simulink model "IBVSstereo"  (Simulink 10.0)
settings: Solver=ode45  StartTime=0.0  StopTime=30.0  RelTol=1e-3  EnableMultiTasking=on
undefined symbols (not defined in the file): coords, get, GetHMatrix, lc, p, rc, T0e_0, T0e_x, T0o, Telc, Terc
libraries: vs x31, simulink x3
settings Model: Creator=bhisma  LastModifiedBy=bhisma
settings DataIOCC: LimitDataPoints=on  SignalLoggingSaveFormat=ModelDataLogs  SignalLoggingName=sigsOut
settings OptimizationCC: BooleanDataType=off  LifeSpan=auto
settings DebuggingCC: SaveWithParameterizedLinksMsg=none  SignalResolutionControl=TryResolveAllWithWarning  MultiTaskDSMMsg=warning  MultiTaskCondExecSysMsg=none  SFUnexpectedBacktrackingDiag=error  SFNoUnconditionalDefaultTransitionDiag=error  SFExecutionAtInitializationDiag=warning  ArithmeticOperatorsInVariantConditions=error
settings HardwareCC: TargetUnknown=on
settings SFSimCC: SimUseLocalCustomCode=on  CustomCodeUndefinedFunction=FilterOut
settings RTWCC: RTWUseLocalCustomCode=on
settings CodeAppCC: StateflowObjectComments=off
settings GRTTargetCC: TargetLangStandard=C99 (ISO)

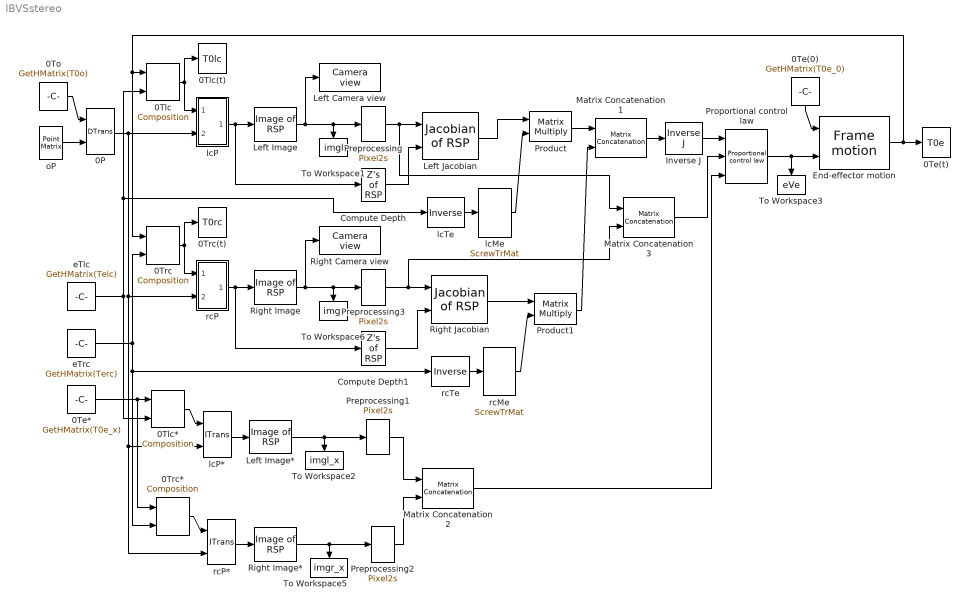
== system IBVSstereo ==
  0P : vs/Features/DTrans  SimViewingDevice=off  DataTypeOverride=UseLocalSettings  MinMaxOverflowLogging=UseLocalSettings
      settings: Permissions=ReadWrite  RTWFcnNameOpts=Auto  RTWFileNameOpts=Auto
  0Te(0) : Constant  Value=GetHMatrix(T0e_0)  VectorParams1D=off
  0Te(t) : ToWorkspace  VariableName=T0e  SaveFormat=Structure With Time  SampleTime=-1
  0Te* : Constant  Value=GetHMatrix(T0e_x)  VectorParams1D=off
  0Tlc : vs/Pose/Composition  SimViewingDevice=off  DataTypeOverride=UseLocalSettings  MinMaxOverflowLogging=UseLocalSettings
      settings: Permissions=ReadWrite  RTWFcnNameOpts=Auto  RTWFileNameOpts=Auto
  0Tlc(t) : ToWorkspace  VariableName=T0lc  SaveFormat=Structure With Time  SampleTime=-1
  0Tlc* : vs/Pose/Composition  SimViewingDevice=off  DataTypeOverride=UseLocalSettings  MinMaxOverflowLogging=UseLocalSettings
      settings: Permissions=ReadWrite  RTWFcnNameOpts=Auto  RTWFileNameOpts=Auto
  0To : Constant  Value=GetHMatrix(T0o)  VectorParams1D=off
  0Trc : vs/Pose/Composition  SimViewingDevice=off  DataTypeOverride=UseLocalSettings  MinMaxOverflowLogging=UseLocalSettings
      settings: Permissions=ReadWrite  RTWFcnNameOpts=Auto  RTWFileNameOpts=Auto
  0Trc(t) : ToWorkspace  VariableName=T0rc  SaveFormat=Structure With Time  SampleTime=-1
  0Trc* : vs/Pose/Composition  SimViewingDevice=off  DataTypeOverride=UseLocalSettings  MinMaxOverflowLogging=UseLocalSettings
      settings: Permissions=ReadWrite  RTWFcnNameOpts=Auto  RTWFileNameOpts=Auto
  Compute Depth : vs/Features/Z's of RSP  SimViewingDevice=off  DataTypeOverride=UseLocalSettings  MinMaxOverflowLogging=UseLocalSettings
      settings: Permissions=ReadWrite  RTWFcnNameOpts=Auto  RTWFileNameOpts=Auto
  Compute Depth1 : vs/Features/Z's of RSP  SimViewingDevice=off  DataTypeOverride=UseLocalSettings  MinMaxOverflowLogging=UseLocalSettings
      settings: Permissions=ReadWrite  RTWFcnNameOpts=Auto  RTWFileNameOpts=Auto
  End-effector motion : vs/Pose/Frame motion  SimViewingDevice=off  DataTypeOverride=UseLocalSettings  MinMaxOverflowLogging=UseLocalSettings
      settings: Permissions=ReadWrite  RTWFcnNameOpts=Auto  RTWFileNameOpts=Auto
  Inverse J : vs/Jacobian/Inverse J  SimViewingDevice=off  DataTypeOverride=UseLocalSettings  MinMaxOverflowLogging=UseLocalSettings
      settings: Permissions=ReadWrite  RTWFcnNameOpts=Auto  RTWFileNameOpts=Auto
  Left Camera view : vs/Camera/Camera view  ms=15  em=normal  umin=0  umax=get(lc,'hres')-1  vmin=0  vmax=get(lc,'vres')-1  st=-1
  Left Image : vs/Camera/Image of RSP  fu=get(lc,'fu')  fv=get(lc,'fv')  u0=get(lc,'u0')  v0=get(lc,'v0')
  Left Image* : vs/Camera/Image of RSP  fu=get(lc,'fu')  fv=get(lc,'fv')  u0=get(lc,'u0')  v0=get(lc,'v0')
  Left Jacobian : vs/Jacobian/Jacobian of RSP  SimViewingDevice=off  DataTypeOverride=UseLocalSettings  MinMaxOverflowLogging=UseLocalSettings
      settings: Permissions=ReadWrite  RTWFcnNameOpts=Auto  RTWFileNameOpts=Auto
  Matrix Concatenation1 : simulink/Math Operations/Matrix Concatenation  numInports=2  catMethod=Vertical
      settings: SourceProductName=Simulink  SourceProductBaseCode=SL
  Matrix Concatenation2 : simulink/Math Operations/Matrix Concatenation  numInports=2  catMethod=Vertical
      settings: SourceProductName=Simulink  SourceProductBaseCode=SL
  Matrix Concatenation3 : simulink/Math Operations/Matrix Concatenation  numInports=2  catMethod=Vertical
      settings: SourceProductName=Simulink  SourceProductBaseCode=SL
  Preprocessing : vs/Jacobian/Pixel2s  fu=get(lc,'fu')  fv=get(lc,'fv')  u0=get(lc,'u0')  v0=get(lc,'v0')
  Preprocessing1 : vs/Jacobian/Pixel2s  fu=get(lc,'fu')  fv=get(lc,'fv')  u0=get(lc,'u0')  v0=get(lc,'v0')
  Preprocessing2 : vs/Jacobian/Pixel2s  fu=get(rc,'fu')  fv=get(rc,'fv')  u0=get(rc,'u0')  v0=get(rc,'v0')
  Preprocessing3 : vs/Jacobian/Pixel2s  fu=get(rc,'fu')  fv=get(rc,'fv')  u0=get(rc,'u0')  v0=get(rc,'v0')
  Product : Product  Multiplication=Matrix(*)  SaturateOnIntegerOverflow=on  InputSameDT=on  OutDataTypeStr=Inherit: Same as first input
  Product1 : Product  Multiplication=Matrix(*)  SaturateOnIntegerOverflow=on  InputSameDT=on  OutDataTypeStr=Inherit: Same as first input
  Proportional control law : vs/Jacobian/Proportional control law  lambda=lambda
  Right Camera view : vs/Camera/Camera view  ms=15  em=normal  umin=0  umax=get(rc,'hres')-1  vmin=0  vmax=get(rc,'vres')-1  st=-1
  Right Image : vs/Camera/Image of RSP  fu=get(rc,'fu')  fv=get(rc,'fv')  u0=get(rc,'u0')  v0=get(rc,'v0')
  Right Image* : vs/Camera/Image of RSP  fu=get(rc,'fu')  fv=get(rc,'fv')  u0=get(rc,'u0')  v0=get(rc,'v0')
  Right Jacobian : vs/Jacobian/Jacobian of RSP  SimViewingDevice=off  DataTypeOverride=UseLocalSettings  MinMaxOverflowLogging=UseLocalSettings
      settings: Permissions=ReadWrite  RTWFcnNameOpts=Auto  RTWFileNameOpts=Auto
  To Workspace1 : ToWorkspace  VariableName=imgl  SaveFormat=Structure With Time  SampleTime=-1
  To Workspace2 : ToWorkspace  VariableName=imgl_x  SaveFormat=Structure With Time  SampleTime=-1
  To Workspace3 : ToWorkspace  VariableName=eVe  SaveFormat=Structure With Time  SampleTime=-1
  To Workspace5 : ToWorkspace  VariableName=imgr_x  SaveFormat=Structure With Time  SampleTime=-1
  To Workspace6 : ToWorkspace  VariableName=imgr  SaveFormat=Structure With Time  SampleTime=-1
  eTlc : Constant  Value=GetHMatrix(Telc)  VectorParams1D=off
  eTrc : Constant  Value=GetHMatrix(Terc)  VectorParams1D=off
  lcMe : vs/Pose/ScrewTrMat  SimViewingDevice=off  DataTypeOverride=UseLocalSettings  MinMaxOverflowLogging=UseLocalSettings
      settings: Permissions=ReadWrite  RTWFcnNameOpts=Auto  RTWFileNameOpts=Auto
  lcP : Subsystem  AncestorBlock=vs/Features/ITrans
  lcP* : vs/Features/ITrans  SimViewingDevice=off  DataTypeOverride=UseLocalSettings  MinMaxOverflowLogging=UseLocalSettings
      settings: Permissions=ReadWrite  RTWFcnNameOpts=Auto  RTWFileNameOpts=Auto
  lcTe : vs/Pose/Inverse  SimViewingDevice=off  DataTypeOverride=UseLocalSettings  MinMaxOverflowLogging=UseLocalSettings
      settings: Permissions=ReadWrite  RTWFcnNameOpts=Auto  RTWFileNameOpts=Auto
  oP : vs/Features/Point Matrix  m=coords(p)
  rcMe : vs/Pose/ScrewTrMat  SimViewingDevice=off  DataTypeOverride=UseLocalSettings  MinMaxOverflowLogging=UseLocalSettings
      settings: Permissions=ReadWrite  RTWFcnNameOpts=Auto  RTWFileNameOpts=Auto
  rcP : Subsystem  AncestorBlock=vs/Features/ITrans
  rcP* : vs/Features/ITrans  SimViewingDevice=off  DataTypeOverride=UseLocalSettings  MinMaxOverflowLogging=UseLocalSettings
      settings: Permissions=ReadWrite  RTWFcnNameOpts=Auto  RTWFileNameOpts=Auto
  rcTe : vs/Pose/Inverse  SimViewingDevice=off  DataTypeOverride=UseLocalSettings  MinMaxOverflowLogging=UseLocalSettings
      settings: Permissions=ReadWrite  RTWFcnNameOpts=Auto  RTWFileNameOpts=Auto
  wires:
  oP/1 -> 0P/2
  lcP/1(bP) -> Compute Depth/1, Left Image/1
  Left Image/1 -> Left Camera view/1, Preprocessing/1, To Workspace1/1
  Preprocessing/1 -> Left Jacobian/1, Matrix Concatenation3/1
  Compute Depth/1 -> Left Jacobian/2
  Inverse J/1 -> Proportional control law/1
  End-effector motion/1 -> 0Te(t)/1, 0Tlc/1, 0Trc/1
  0Te*/1 -> 0Tlc*/1, 0Trc*/1
  lcP*/1 -> Left Image*/1
  0Te(0)/1 -> End-effector motion/1
  0To/1 -> 0P/1
  0P/1 -> lcP/2(aP), lcP*/2, rcP*/2, rcP/2(aP)
  Proportional control law/1 -> End-effector motion/2, To Workspace3/1
  Left Image*/1 -> Preprocessing1/1, To Workspace2/1
  0Tlc/1 -> lcP/1(aTb), 0Tlc(t)/1
  eTlc/1 -> 0Tlc*/2, 0Tlc/2, lcTe/1
  0Tlc*/1 -> lcP*/1
  rcP*/1 -> Right Image*/1
  Right Image*/1 -> Preprocessing2/1, To Workspace5/1
  0Trc*/1 -> rcP*/1
  eTrc/1 -> 0Trc/2, 0Trc*/2, rcTe/1
  rcP/1(bP) -> Compute Depth1/1, Right Image/1
  Right Image/1 -> Right Camera view/1, Preprocessing3/1, To Workspace6/1
  Preprocessing3/1 -> Right Jacobian/1, Matrix Concatenation3/2
  Compute Depth1/1 -> Right Jacobian/2
  0Trc/1 -> rcP/1(aTb), 0Trc(t)/1
  lcTe/1 -> lcMe/1
  Product/1 -> Matrix Concatenation1/1
  Matrix Concatenation1/1 -> Inverse J/1
  Left Jacobian/1 -> Product/1
  lcMe/1 -> Product/2
  rcTe/1 -> rcMe/1
  rcMe/1 -> Product1/2
  Right Jacobian/1 -> Product1/1
  Product1/1 -> Matrix Concatenation1/2
  Preprocessing1/1 -> Matrix Concatenation2/1
  Preprocessing2/1 -> Matrix Concatenation2/2
  Matrix Concatenation3/1 -> Proportional control law/2
  Matrix Concatenation2/1 -> Proportional control law/3

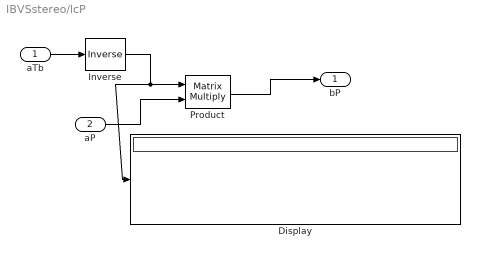
== system IBVSstereo/lcP ==
  aTb : Inport
  aP : Inport  Port=2
  Display : Display
  Inverse : vs/Pose/Inverse  SimViewingDevice=off  DataTypeOverride=UseLocalSettings  MinMaxOverflowLogging=UseLocalSettings
      settings: Permissions=ReadWrite  RTWFcnNameOpts=Auto  RTWFileNameOpts=Auto
  Product : Product  Multiplication=Matrix(*)  SaturateOnIntegerOverflow=on  InputSameDT=on  OutDataTypeStr=Inherit: Same as first input
  bP : Outport
  wires:
  Inverse/1 -> Product/1, Display/1
  aTb/1 -> Inverse/1
  Product/1 -> bP/1
  aP/1 -> Product/2

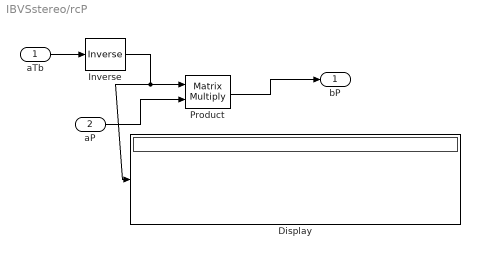
== system IBVSstereo/rcP ==
  aTb : Inport
  aP : Inport  Port=2
  Display : Display
  Inverse : vs/Pose/Inverse  SimViewingDevice=off  DataTypeOverride=UseLocalSettings  MinMaxOverflowLogging=UseLocalSettings
      settings: Permissions=ReadWrite  RTWFcnNameOpts=Auto  RTWFileNameOpts=Auto
  Product : Product  Multiplication=Matrix(*)  SaturateOnIntegerOverflow=on  InputSameDT=on  OutDataTypeStr=Inherit: Same as first input
  bP : Outport
  wires:
  Inverse/1 -> Product/1, Display/1
  aTb/1 -> Inverse/1
  Product/1 -> bP/1
  aP/1 -> Product/2
